simulink model "Capstone"  (R2021a)
settings: Solver=VariableStepAuto  StartTime=0.0  StopTime=10.0  RelTol=1e-3
settings Model: Creator=davidedelson  LastModifiedBy=TJ Perusek
settings SolverCC: AlgebraicLoopSolver=TrustRegion
settings DebuggingCC: SFMachineParentedDataDiag=warning

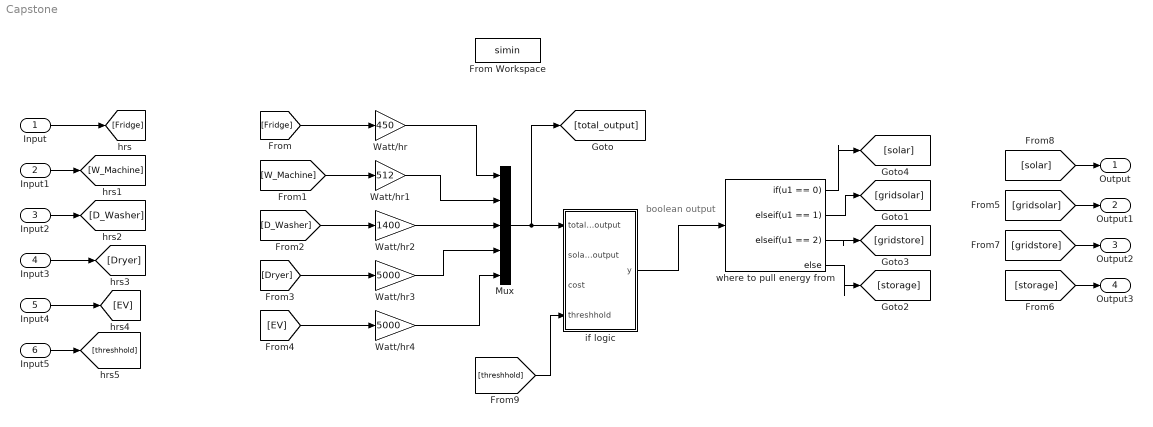
== system Capstone ==
  note: boolean output
  Input : Inport
  Input1 : Inport  Port=2
  Input2 : Inport  Port=3
  Input3 : Inport  Port=4
  Input4 : Inport  Port=5
  Input5 : Inport  Port=6
  From Workspace : FromWorkspace  VariableName=simin
  Mux : Mux  Inputs=5
  Watt/hr : Gain  Gain=450
  Watt/hr1 : Gain  Gain=512
  Watt/hr2 : Gain  Gain=1400
  Watt/hr3 : Gain  Gain=5000
  Watt/hr4 : Gain  Gain=5000
  if logic : MATLAB Function  TreatAsAtomicUnit=on
  where to pull energy from : If  IfExpression=u1 == 0  ElseIfExpressions=u1 == 1, u1 == 2
  Output : Outport
  Output1 : Outport  Port=2
  Output2 : Outport  Port=3
  Output3 : Outport  Port=4
  wires:
  [Fridge] -> Watt/hr/1
  [W_Machine] -> Watt/hr1/1
  [D_Washer] -> Watt/hr2/1
  [Dryer] -> Watt/hr3/1
  [EV] -> Watt/hr4/1
  Input/1 -> [Fridge]
  Input1/1 -> [W_Machine]
  Input3/1 -> [Dryer]
  Input2/1 -> [D_Washer]
  Input4/1 -> [EV]
  Mux/1 -> [total_output], if logic/1(total_output)
  Watt/hr/1 -> Mux/1
  Watt/hr1/1 -> Mux/2
  Watt/hr2/1 -> Mux/3
  Watt/hr3/1 -> Mux/4
  Watt/hr4/1 -> Mux/5
  if logic/1(y) -> where to pull energy from/1
  where to pull energy from/1 -> [solar]
  where to pull energy from/4 -> [storage]
  [gridsolar] -> Output1/1
  [gridstore] -> Output2/1
  [storage] -> Output3/1
  where to pull energy from/3 -> [gridstore]
  where to pull energy from/2 -> [gridsolar]
  [solar] -> Output/1
  Input5/1 -> [threshhold]
  [threshhold] -> if logic/4(threshhold)

== matlab function Capstone/if logic ==
  data: total_output input; y output; solar_output input; cost input; threshhold input
function y = fcn(total_output, solar_output, cost, threshhold)

if (solar_output > total_output)
    decision_output = 0;
if (total_output > solar_output)
    if (cost > threshhold && has_storage == false)
        decision_output = 1;
    elseif (cost > threshhold && has_storage == true)
        decision_output = 3;
    elseif (cost < threshhold && has_storage == false)
        decision_output = 1;
    else (cost < threshhold && has_storage == true)
        decision_output = 2;
        
% offpeak = 10pm-6am
% midpeak = 6am-2pm && 7p-10pm
% peak= 2pm-7pm;

if(datetime('now'))
    cost = ;
y = decision_output;
